simulink model "ScenarioLib"  (Simulink 7.8)
settings: Solver=ode45  StartTime=0.0  StopTime=10.0  RelTol=1e-3
undefined symbols (not defined in the file): sigbuilder_block
libraries: simulink x6, instrumentlib x4, utility x1, dspnetwork x1
settings Model: Creator=Zsolt  LastModifiedBy=jscott
settings DebuggingCC: FcnCallInpInsideContextMsg=Use local settings
settings HardwareCC: TargetIntDivRoundTo=Zero  TargetEndianess=LittleEndian  TargetHWDeviceType=MATLAB Host  ProdEqTarget=off
settings RTWCC: SystemTargetFile=rsim.tlc  TemplateMakefile=rsim_default_tmf  Description=Rapid Simulation Target  ProcessScript=rsim_make_rtw_hook
settings RSimTargetCC: TargetFunctionLibrary=ANSI_C  ERTMultiwordTypeDef=System defined  CodeExecutionProfiling=off  ERTMultiwordLength=256  IsPILTarget=off  EnableShiftOperators=on  PortableWordSizes=off

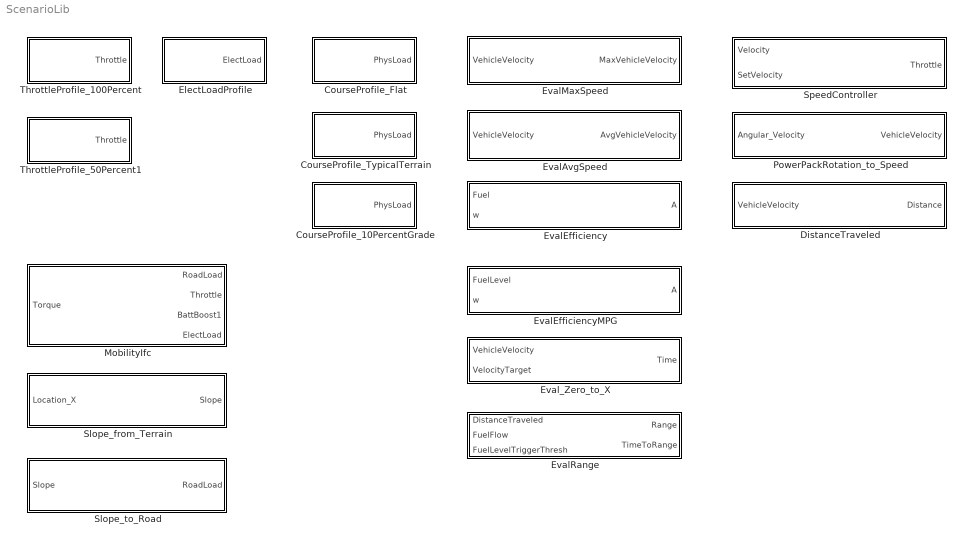
== system ScenarioLib ==
  CourseProfile_10PercentGrade : Subsystem
  CourseProfile_Flat : Subsystem
  CourseProfile_TypicalTerrain : Subsystem
  DistanceTraveled : Subsystem
  ElectLoadProfile : Subsystem
  EvalAvgSpeed : Subsystem
  EvalEfficiency : Subsystem
  EvalEfficiencyMPG : Subsystem
  EvalMaxSpeed : Subsystem
  EvalRange : Subsystem
  Eval_Zero_to_X : Subsystem
  MobilityIfc : Subsystem
  PowerPackRotation_to_Speed : Subsystem
  Slope_from_Terrain : Subsystem
  Slope_to_Road : Subsystem
  SpeedController : Subsystem
  ThrottleProfile_100Percent : Subsystem
  ThrottleProfile_50Percent1 : Subsystem

== system ScenarioLib/CourseProfile_10PercentGrade ==
  Flat : Subsystem  Tag=STV Subsys  LoadFcn=sigbuilder_block('load');  StartFcn=sigbuilder_block('start');  StopFcn=sigbuilder_block('stop');  ClipboardFcn=sigbuilder_block('clipboard');  mask(Sigbuilder block){}
      mask help: Create and generate interchangeable groups of signals whose waveforms are piecewise linear.
      mask init:
      | if ~strcmp(get_param(bdroot(gcbh),'SimulationStatus'),'stopped') tuvar = sigbuilder_block('maskInit'); end
      settings: CopyFcn=sigbuilder_block('copy');  DeleteFcn=sigbuilder_block('delete');  ModelCloseFcn=sigbuilder_block('modelClose');  PreSaveFcn=sigbuilder_block('preSave');  NameChangeFcn=sigbuilder_block('namechange');  OpenFcn=sigbuilder_block('open',[62.6897 69.5172 970.759 504 ]);  CloseFcn=sigbuilder_block('close');
      mask Display: plot(0,0,100,100,[10,10,40,40,10],[80,20,20,80,80],[40,10],[50,50], [40,27,10],[65,72,56],[40,25,25,10],[28,28,43,43]);
  PhysLoad : Outport
  wires:
  Flat/1(PhysLoad) -> PhysLoad/1

== system ScenarioLib/CourseProfile_Flat ==
  Flat : Subsystem  Tag=STV Subsys  LoadFcn=sigbuilder_block('load');  StartFcn=sigbuilder_block('start');  StopFcn=sigbuilder_block('stop');  ClipboardFcn=sigbuilder_block('clipboard');  mask(Sigbuilder block){}
      mask help: Create and generate interchangeable groups of signals whose waveforms are piecewise linear.
      mask init:
      | if ~strcmp(get_param(bdroot(gcbh),'SimulationStatus'),'stopped') tuvar = sigbuilder_block('maskInit'); end
      settings: CopyFcn=sigbuilder_block('copy');  DeleteFcn=sigbuilder_block('delete');  ModelCloseFcn=sigbuilder_block('modelClose');  PreSaveFcn=sigbuilder_block('preSave');  NameChangeFcn=sigbuilder_block('namechange');  OpenFcn=sigbuilder_block('open',[62.6897 69.5172 970.759 504 ]);  CloseFcn=sigbuilder_block('close');
      mask Display: plot(0,0,100,100,[10,10,40,40,10],[80,20,20,80,80],[40,10],[50,50], [40,27,10],[65,72,56],[40,25,25,10],[28,28,43,43]);
  PhysLoad : Outport
  wires:
  Flat/1(PhysLoad) -> PhysLoad/1

== system ScenarioLib/CourseProfile_TypicalTerrain ==
  TypicalTerrain : Subsystem  Tag=STV Subsys  LoadFcn=sigbuilder_block('load');  StartFcn=sigbuilder_block('start');  StopFcn=sigbuilder_block('stop');  ClipboardFcn=sigbuilder_block('clipboard');  mask(Sigbuilder block){}
      mask help: Create and generate interchangeable groups of signals whose waveforms are piecewise linear.
      mask init:
      | if ~strcmp(get_param(bdroot(gcbh),'SimulationStatus'),'stopped') tuvar = sigbuilder_block('maskInit'); end
      settings: CopyFcn=sigbuilder_block('copy');  DeleteFcn=sigbuilder_block('delete');  ModelCloseFcn=sigbuilder_block('modelClose');  PreSaveFcn=sigbuilder_block('preSave');  NameChangeFcn=sigbuilder_block('namechange');  OpenFcn=sigbuilder_block('open',[164.483 27.3103 970.138 504 ]);  CloseFcn=sigbuilder_block('close');
      mask Display: plot(0,0,100,100,[10,10,40,40,10],[80,20,20,80,80],[40,10],[50,50], [40,27,10],[65,72,56],[40,25,25,10],[28,28,43,43]);
  PhysLoad : Outport
  wires:
  TypicalTerrain/1(PhysLoad) -> PhysLoad/1

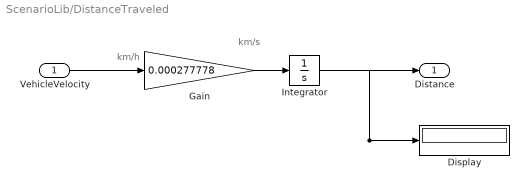
== system ScenarioLib/DistanceTraveled ==
  note: km/h
  note: km/s
  VehicleVelocity : Inport
  Display : Display
  Gain : Gain  Gain=0.000277778
  Integrator : Integrator
  Distance : Outport
  wires:
  VehicleVelocity/1 -> Gain/1
  Integrator/1 -> Distance/1, Display/1
  Gain/1 -> Integrator/1

== system ScenarioLib/ElectLoadProfile ==
  Elect_Load_Driver : Subsystem  Tag=STV Subsys  LoadFcn=sigbuilder_block('load');  StartFcn=sigbuilder_block('start');  StopFcn=sigbuilder_block('stop');  ClipboardFcn=sigbuilder_block('clipboard');  mask(Sigbuilder block){}
      mask help: Create and generate interchangeable groups of signals whose waveforms are piecewise linear.
      mask init:
      | if ~strcmp(get_param(bdroot(gcbh),'SimulationStatus'),'stopped') tuvar = sigbuilder_block('maskInit'); end
      settings: CopyFcn=sigbuilder_block('copy');  DeleteFcn=sigbuilder_block('delete');  ModelCloseFcn=sigbuilder_block('modelClose');  PreSaveFcn=sigbuilder_block('preSave');  NameChangeFcn=sigbuilder_block('namechange');  OpenFcn=sigbuilder_block('open',[164.483 24.8276 970.138 502.759 ]);  CloseFcn=sigbuilder_block('close');
      mask Display: plot(0,0,100,100,[10,10,40,40,10],[80,20,20,80,80],[40,10],[50,50], [40,27,10],[65,72,56],[40,25,25,10],[28,28,43,43]);
  ElectLoad : Outport
  wires:
  Elect_Load_Driver/1(Elect Load) -> ElectLoad/1

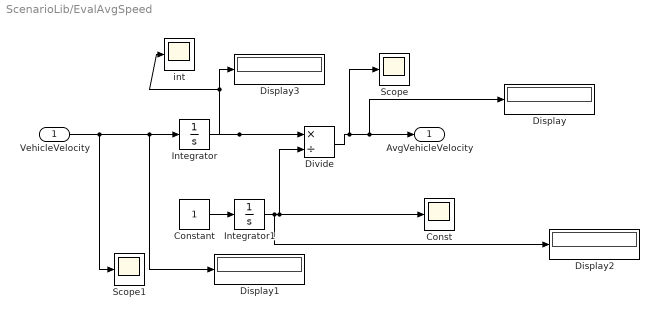
== system ScenarioLib/EvalAvgSpeed ==
  VehicleVelocity : Inport
  Const : Scope
      settings: YMin=250  YMax=4250
  Constant : Constant
  Display{,1..3} (4 alike) : Display
  Divide : Product  Inputs=*/
  Integrator : Integrator
  Integrator1 : Integrator  InitialCondition=0.001
  Scope : Scope
      settings: YMin=250  YMax=4250  SaveName=ScopeData2
  Scope1 : Scope
      settings: YMin=250  YMax=4250  SaveName=ScopeData3
  int : Scope
      settings: YMin=250  YMax=4250  SaveName=ScopeData4
  AvgVehicleVelocity : Outport
  wires:
  Divide/1 -> Scope/1, AvgVehicleVelocity/1, Display/1
  VehicleVelocity/1 -> Scope1/1, Display1/1, Integrator/1
  Constant/1 -> Integrator1/1
  Integrator/1 -> Divide/1, Display3/1, int/1
  Integrator1/1 -> Display2/1, Divide/2, Const/1

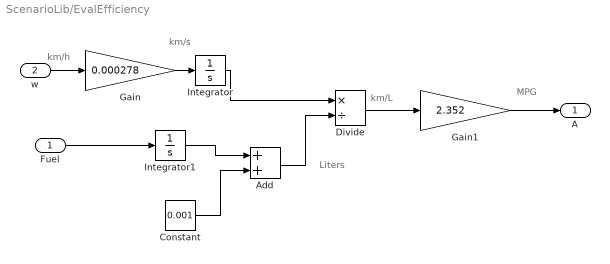
== system ScenarioLib/EvalEfficiency ==
  note: km/h
  note: km/s
  note: Liters
  note: km/L
  note: MPG
  Fuel : Inport
  w : Inport  Port=2
  Add : Sum
  Constant : Constant  Value=0.001
  Divide : Product  Inputs=*/
  Gain : Gain  Gain=0.000278
  Gain1 : Gain  Gain=2.352
  Integrator : Integrator
  Integrator1 : Integrator
  A : Outport
  wires:
  Integrator1/1 -> Add/1
  Constant/1 -> Add/2
  Fuel/1 -> Integrator1/1
  Add/1 -> Divide/2
  Integrator/1 -> Divide/1
  w/1 -> Gain/1
  Gain/1 -> Integrator/1
  Gain1/1 -> A/1
  Divide/1 -> Gain1/1

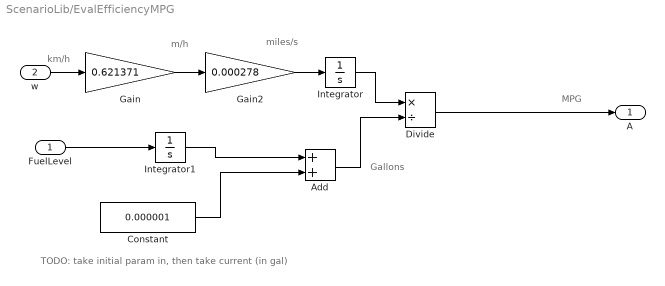
== system ScenarioLib/EvalEfficiencyMPG ==
  note: km/h
  note: m/h
  note: Gallons
  note: MPG
  note: TODO: take initial param in, then take current (in gal)
  note: miles/s
  FuelLevel : Inport
  w : Inport  Port=2
  Add : Sum
  Constant : Constant  Value=0.000001
  Divide : Product  Inputs=*/
  Gain : Gain  Gain=0.621371
  Gain2 : Gain  Gain=0.000278
  Integrator : Integrator
  Integrator1 : Integrator
  A : Outport
  wires:
  Integrator1/1 -> Add/1
  Constant/1 -> Add/2
  FuelLevel/1 -> Integrator1/1
  Add/1 -> Divide/2
  Integrator/1 -> Divide/1
  w/1 -> Gain/1
  Divide/1 -> A/1
  Gain2/1 -> Integrator/1
  Gain/1 -> Gain2/1

== system ScenarioLib/EvalMaxSpeed ==
  VehicleVelocity : Inport
  MinMax Running Resettable : simulink/Math Operations/MinMax Running Resettable  Function=max  vinit=0.0
  MaxVehicleVelocity : Outport
  wires:
  VehicleVelocity/1 -> MinMax Running Resettable/1
  MinMax Running Resettable/1 -> MaxVehicleVelocity/1

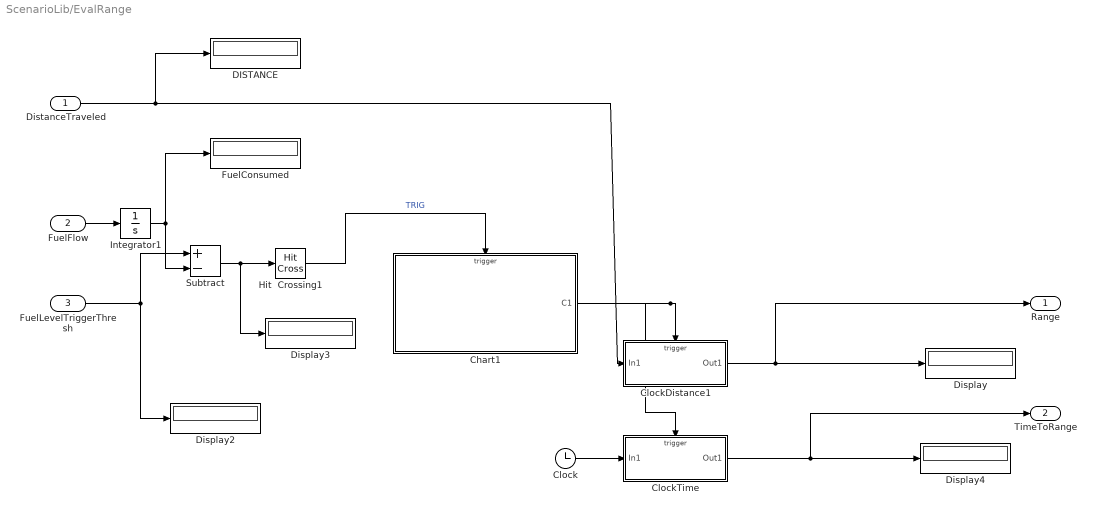
== system ScenarioLib/EvalRange ==
  DistanceTraveled : Inport
  FuelFlow : Inport  Port=2
  FuelLevelTriggerThresh : Inport  Port=3
  Chart1 : Stateflow chart  TreatAsAtomicUnit=on
  Clock : Clock
  ClockDistance1 : Subsystem  TreatAsAtomicUnit=on
  ClockTime : Subsystem  TreatAsAtomicUnit=on
  DISTANCE : Display
  Display{,2..4} (4 alike) : Display
  FuelConsumed : Display
  Hit  Crossing1 : HitCross  HitCrossingDirection=falling  ZeroCross=off
  Integrator1 : Integrator
  Subtract : Sum  Inputs=+-
  Range : Outport
  TimeToRange : Outport  Port=2
  wires:
  DistanceTraveled/1 -> ClockDistance1/1(In1), DISTANCE/1
  Hit  Crossing1/1 -> Chart1/Trigger  "TRIG"
  Chart1/1(C1) -> ClockDistance1/Trigger, ClockTime/Trigger
  ClockDistance1/1(Out1) -> Range/1, Display/1
  FuelFlow/1 -> Integrator1/1
  FuelLevelTriggerThresh/1 -> Display2/1, Subtract/1
  Subtract/1 -> Hit  Crossing1/1, Display3/1
  Clock/1 -> ClockTime/1(In1)
  ClockTime/1(Out1) -> TimeToRange/1, Display4/1
  Integrator1/1 -> FuelConsumed/1, Subtract/2

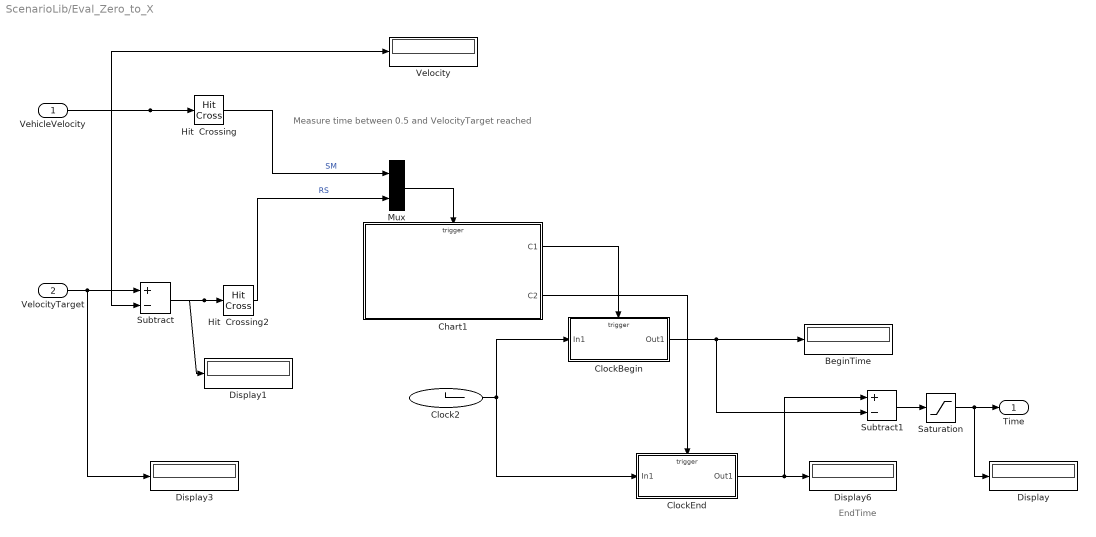
== system ScenarioLib/Eval_Zero_to_X ==
  note: EndTime
  note: Measure time between 0.5 and VelocityTarget reached
  VehicleVelocity : Inport
  VelocityTarget : Inport  Port=2
  BeginTime : Display
  Chart1 : Stateflow chart  TreatAsAtomicUnit=on
  Clock2 : Clock
  ClockBegin : Subsystem  TreatAsAtomicUnit=on
  ClockEnd : Subsystem  TreatAsAtomicUnit=on
  Display{,1,3,6} (4 alike) : Display
  Hit  Crossing : HitCross  HitCrossingOffset=0.5  HitCrossingDirection=rising
  Hit  Crossing2 : HitCross  HitCrossingDirection=falling  ZeroCross=off
  Mux : Mux  Inputs=2
  Saturation : Saturate  UpperLimit=10000000  LowerLimit=0.0  ZeroCross=off
  Subtract : Sum  Inputs=+-
  Subtract1 : Sum  Inputs=+-
  Velocity : Display
  Time : Outport
  wires:
  ClockBegin/1(Out1) -> BeginTime/1, Subtract1/2
  ClockEnd/1(Out1) -> Display6/1, Subtract1/1
  Chart1/2(C2) -> ClockEnd/Trigger
  Subtract/1 -> Display1/1, Hit  Crossing2/1
  VelocityTarget/1 -> Subtract/1, Display3/1
  Chart1/1(C1) -> ClockBegin/Trigger
  Hit  Crossing2/1 -> Mux/2  "RS"
  Hit  Crossing/1 -> Mux/1  "SM"
  Clock2/1 -> ClockBegin/1(In1), ClockEnd/1(In1)
  Mux/1 -> Chart1/Trigger
  VehicleVelocity/1 -> Hit  Crossing/1, Subtract/2, Velocity/1
  Subtract1/1 -> Saturation/1
  Saturation/1 -> Time/1, Display/1

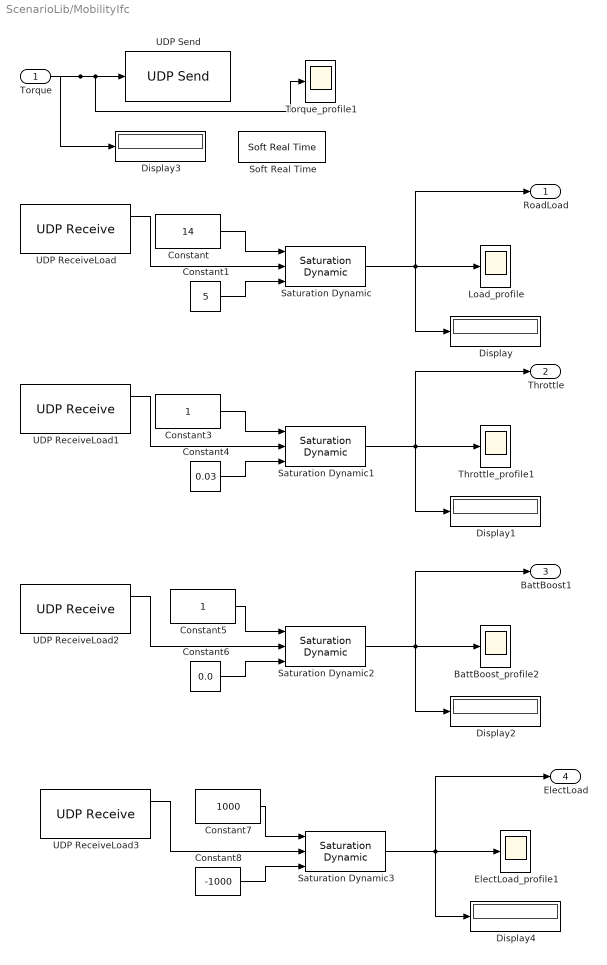
== system ScenarioLib/MobilityIfc ==
  Torque : Inport
  BattBoost_profile2 : Scope
      settings: TimeRange=500  YMin=0  YMax=150000  SaveName=ScopeData3
  Constant : Constant  Value=14
  Constant1 : Constant  Value=5
  Constant3 : Constant
  Constant4 : Constant  Value=0.03
  Constant5 : Constant
  Constant6 : Constant  Value=0.0
  Constant7 : Constant  Value=1000
  Constant8 : Constant  Value=-1000
  Display{,1..4} (5 alike) : Display
  ElectLoad_profile1 : Scope
      settings: TimeRange=500  YMin=0  YMax=150000  SaveName=ScopeData5
  Load_profile : Scope
      settings: TimeRange=500  YMin=0  YMax=150000
  Saturation Dynamic{,1..3} (4 alike) : simulink/Discontinuities/Saturation Dynamic  OutMin=[]  OutMax=[]  OutDataTypeStr=Inherit: Same as second input  OutDataType=fixdt(1, 16)  OutScaling=2^-10  DoSatur=off
  Soft Real Time : utility/Soft Real Time  x=1
  Throttle_profile1 : Scope
      settings: TimeRange=500  YMin=0  YMax=150000
  Torque_profile1 : Scope
      settings: TimeRange=100  YMin=0  YMax=150000  SaveName=ScopeData4
  UDP ReceiveLoad : instrumentlib/UDP Receive  Host=localhost  Port=9090  LocalPort=8090  DataSize=[1 1]  EnableBlockingMode=off  Timeout=10  SampleTime=0.08  DataType=double  ByteOrder=LittleEndian
  UDP ReceiveLoad1 : instrumentlib/UDP Receive  Host=localhost  Port=9090  LocalPort=8092  DataSize=[1 1]  EnableBlockingMode=off  Timeout=10  SampleTime=0.08  DataType=double  ByteOrder=LittleEndian
  UDP ReceiveLoad2 : instrumentlib/UDP Receive  Host=localhost  Port=9090  LocalPort=8093  DataSize=[1 1]  EnableBlockingMode=off  Timeout=10  SampleTime=0.08  DataType=double  ByteOrder=LittleEndian
  UDP ReceiveLoad3 : instrumentlib/UDP Receive  Host=localhost  Port=9090  LocalPort=8098  DataSize=[1 1]  EnableBlockingMode=off  Timeout=10  SampleTime=0.08  DataType=double  ByteOrder=LittleEndian
  UDP Send : dspnetwork/UDP Send  remoteURL='127.0.0.1'  remotePort=8094  localURL='0.0.0.0'  localPortSource=Automatically determine  localPort=-1  sampletime=-1  separateLengthPort=0
  RoadLoad : Outport
  Throttle : Outport  Port=2
  BattBoost1 : Outport  Port=3
  ElectLoad : Outport  Port=4
  wires:
  Constant/1 -> Saturation Dynamic/1
  Constant1/1 -> Saturation Dynamic/3
  Saturation Dynamic/1 -> Load_profile/1, Display/1, RoadLoad/1
  UDP ReceiveLoad/1 -> Saturation Dynamic/2
  Constant3/1 -> Saturation Dynamic1/1
  Constant4/1 -> Saturation Dynamic1/3
  Saturation Dynamic1/1 -> Throttle_profile1/1, Display1/1, Throttle/1
  UDP ReceiveLoad1/1 -> Saturation Dynamic1/2
  Constant5/1 -> Saturation Dynamic2/1
  Constant6/1 -> Saturation Dynamic2/3
  Saturation Dynamic2/1 -> BattBoost_profile2/1, Display2/1, BattBoost1/1
  UDP ReceiveLoad2/1 -> Saturation Dynamic2/2
  Torque/1 -> UDP Send/1, Torque_profile1/1, Display3/1
  Constant7/1 -> Saturation Dynamic3/1
  Constant8/1 -> Saturation Dynamic3/3
  Saturation Dynamic3/1 -> ElectLoad_profile1/1, Display4/1, ElectLoad/1
  UDP ReceiveLoad3/1 -> Saturation Dynamic3/2

== system ScenarioLib/PowerPackRotation_to_Speed ==
  Angular_Velocity : Inport
  Gain : Gain  Gain=0.3
  VehicleVelocity : Outport
  wires:
  Gain/1 -> VehicleVelocity/1
  Angular_Velocity/1 -> Gain/1

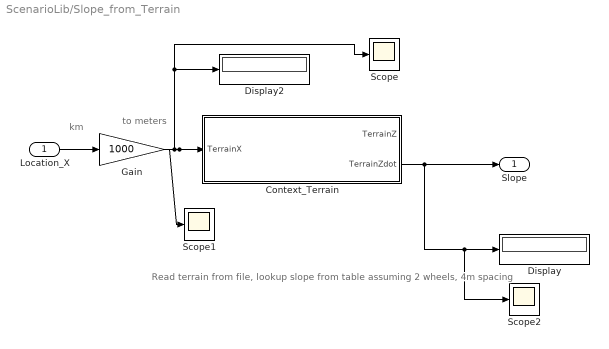
== system ScenarioLib/Slope_from_Terrain ==
  note: Read terrain from file, lookup slope from table
      |  assuming 2 wheels, 4m spacing
  note: km
  note: to meters
  Location_X : Inport
  Context_Terrain : Subsystem  mask(Context Model Terrain for Fuel Efficiency){TerrainFilename=terrain.txt, Use_Old_Terrain=off, Input0_Height=0, Input_QueryDist=off, Output_Height_CkBx=on, Output_Slope_CkBx=on, TerrainLength=20000}
      mask prompts: TerrainFilename "Terrain Filename"; Use_Old_Terrain "Use Existing Terrain"; Input0_Height "Initial Terrain Height"; Input_QueryDist "Query with Distance Traveled"; Output_Height_CkBx "Height_Output"; Output_Slope_CkBx "Slope_Output"; TerrainLength "Desired Terrain Length"
      mask help: Generates a sample terrain from a Probability Density Function fit of US CONUS DEM data. The DEM data was sampled at 90 meter increments, consequently the data establishes long wavelength changes in slope suitable for the study of gross elevation changes on a system design.
      mask init:
      | ThisBlock = gcb;
      | % verify the existence of terrain file
      | if and(strcmp(Use_Old_Terrain, 'off'), ...
      |         ~exist(TerrainFilename, 'file'))
      |     msgbox(['Terrain filename: ', TerrainFilename, ...
      |         ' does not exist. Setting "Use Existing ', ...
      |         'Terrain" checkbox to create new instance', ...
      |         '.  Remember to un-check it after this run.']);
      |     set_param(ThisBlock, 'Use_Old_Terrain', 'off');
      | end
      | % test for terrain synthesis
      | if strcmp(Use_Old_Terrain, 'on')
      |     % load up the existing terrain data
      |     x = load(TerrainFilename, 'ascii');
      |     % terrain data is stored in orthogonal coordinates
      |     % calculate the slope data and load it up
      |     SignedSlope = [diff(x(:,2))./diff(x(:,1)),0];
      | else
      |     % generate some new terrain
      |     npts = ceil(TerrainLength/92/2)*2;
      |     x = zeros(npts,2);
      |     x(:,1) = [0:92:(npts-1)*92]'; % distance in meters
      |     % form a slope array
      |     Slope = 0.037*(log(rand(npts,1))+log(rand(npts,1)));
      |     SignedSlope = sign(rand(npts,1)-0.5).*Slope;
      |     % Form the elevation array
      |     Elevation = [0; diff(x(:,1))].*SignedSlope;
      |     x(:,2) = cumsum(Elevation)'; % distance in meters
      |     % save the synthesized terrain
      |     save(TerrainFilename, 'x', '-ascii')
      | end
      | % adjust for terrain query method
      | if strcmp(Input_QueryDist, 'on')
      |     % set for distance traveled
      |     terrain_in = [0, cumsum(sqrt(diff(x(:,1)).^2 + ...
      |         diff(x(:,2)).^2))];
      | else
      |     terrain_in = x(:,1)';
      | end
      | terrain_out = x(:,2)';
      | % load up the terrain data into the lookup tables
      | set_param([ThisBlock, '/Terrain Height'], ...
      |     'InputValues', ['[', num2str(terrain_in), ']'], ...
      |     'OutputValues', ['[', num2str(terrain_out), ']']);
      | set_param([ThisBlock, '/Terrain Heightdot'], ...
      |     'InputValues', ['[', num2str(terrain_in), ']'], ...
      |     'OutputValues', ['[', num2str(SignedSlope(2:end)'), ' 0]']);
      mask Help:
      | Copyright (c) 2012, BAE Systems.
      | Developed with the sponsorship of the Defense Advanced Research Projects Agency (DARPA).
      | 
      | Permission is hereby granted, free of charge, to any person obtaining a copy of this data,
      | including any software or models in source or binary form, as well as any drawings,
      | specifications, and documentation (collectively "the Data"), to deal in the Data without restriction,
      | including without limitation the rights to use, copy, modify, merge, publish, distribute, sublicense,
      | and/or sell copies of the Data, and to permit persons to whom the Data is furnished to do so,
      | subject to the following conditions:
      | 
      | The above copyright notice and this permission notice shall be included in all copies or substantial
      | portions of the Data.
      | 
      | THE DATA IS PROVIDED "AS IS", WITHOUT WARRANTY OF ANY KIND, EXPRESS OR IMPLIED, INCLUDING
      | BUT NOT LIMITED TO THE WARRANTIES OF MERCHANTABILITY, FITNESS FOR A PARTICULAR PURPOSE
      | AND NONINFRINGEMENT. IN NO EVENT SHALL THE AUTHORS, SPONSORS, DEVELOPERS, CONTRIBUTORS,
      | OR COPYRIGHT HOLDERS BE LIABLE FOR ANY CLAIM, DAMAGES OR OTHER LIABILITY, WHETHER IN AN
      | ACTION OF CONTRACT, TORT OR OTHERWISE, ARISING FROM, OUT OF OR IN CONNECTION WITH THE
      | DATA OR THE USE OR OTHER DEALINGS IN THE DATA.
      mask CallbackString:
      | ThisBlock = gcb;
      | Use_Old_Terrain = get_param(ThisBlock, 'Use_Old_Terrain');
      | TerrainFilename = get_param(ThisBlock, 'TerrainFilename');
      | % file must exist for terrain use
      | if strcmp(Use_Old_Terrain,'on')
      |     if ~exist(TerrainFilename, 'file')
      |         msgbox(['Terrain filename: ', TerrainFilename, ...
      |             ' does not exist. Setting "Use Existing ', ...
      |             'Terrain" checkbox to create new instance', ...
      |             '.  Remember to un-check it after this run.']);
      |         % uncheck the Use Old Terrain chkbox
      |         set_param(ThisBlock, 'Use_Old_Terrain', 'off');
      |     end
      | end|ThisBlock = gcb;
      | Use_Old_Terrain = get_param(ThisBlock, 'Use_Old_Terrain');
      | TerrainFilename = get_param(ThisBlock, 'TerrainFilename');
      | % file must exist for terrain use
      | if strcmp(Use_Old_Terrain,'on')
      |     if ~exist(TerrainFilename, 'file')
      |         msgbox(['Terrain filename: ', TerrainFilename, ...
      |             ' does not exist. Setting "Use Existing ', ...
      |             'Terrain" checkbox to create new instance', ...
      |             '.  Change "Terrain Filename" to existing', ...
      |             ' file before setting this checkbox.']);
      |         % uncheck the Use Old Terrain chkbox
      |         set_param(ThisBlock, 'Use_Old_Terrain', 'off');
      |     else
      |         % load up the terrain file and change the length parameter
      |         tmp = load(TerrainFilename, 'ascii');
      |         TerrainLength = max(tmp(:,1));
      |         % change the terrain length parameter
      |         set_param(ThisBlock, 'TerrainLength', num2str(TerrainLength));
      |     end
      | end|ThisBlock = gcb;
      | Input0_Height = get_param(ThisBlock, 'Input0_Height');
      | % set the constant offset block
      | set_param([ThisBlock, '/Ref_Height'], 'Value', num2str(Input0_Height));||ThisBlock = gcb;
      | Output_Slope_CkBx = get_param(ThisBlock, 'Output_Slope_CkBx');
      | Output_Height_CkBx = get_param(ThisBlock, 'Output_Height_CkBx');
      | % check what number to use for the output port
      | if strcmp(Output_Height_CkBx, 'on')
      |     if strcmp(Output_Slope_CkBx, 'on')
      |         % set the output port number to 2
      |         set_param([ThisBlock, '/TerrainZdot'], ...
      |             'Port', '2');
      |     end
      |     % replace with output block
      |     replace_block([ThisBlock, '/TerrainZ'], ...
      |         'Terminator', 'built-in/Outport', ...
      |         'noprompt')
      | else
      |     % replace with Terminator
      |     replace_block([ThisBlock, '/TerrainZ'], ...
      |         'Outport', 'built-in/Terminator', ...
      |         'noprompt')
      | end
      | |ThisBlock = gcb;
      | Output_Slope_CkBx = get_param(ThisBlock, 'Output_Slope_CkBx');
      | Output_Height_CkBx = get_param(ThisBlock, 'Output_Height_CkBx');
      | % check what number to use for the output port
      | if strcmp(Output_Height_CkBx, 'on')
      |     % set the output port number to 2
      |     SlopePortNum = '2';
      | else
      |     SlopePortNum = '1';
      | end
      | % set or add the appropriate outputs
      | if strcmp(Output_Slope_CkBx, 'on')
      |     % replace with output block
      |     replace_block([ThisBlock, '/TerrainZdot'], ...
      |         'Terminator', 'built-in/Outport', ...
      |         'noprompt')
      |     set_param([ThisBlock, '/TerrainZdot'], ...
      |         'Port', SlopePortNum);
      | else
      |     % replace with Terminator
      |     replace_block([ThisBlock, '/TerrainZdot'], ...
      |         'Outport', 'built-in/Terminator', ...
      |         'noprompt')
      | end|ThisBlock = gcb;
      | TerrainLength = get_param(ThisBlock, 'TerrainLength');
      | % verify that the length is positive
      | if str2num(TerrainLength)<=0
      |     msgbox(['Desired terrain length needs to be greater than zero.  ', ...
      |         'Setting the value to 1000 meters.']);
      |     set_param(ThisBlock, 'TerrainLength', num2str(1000));
      | end
      mask TabNameString: Primary,Primary,Primary,Set-up,Set-up,Set-up,Set-up
  Display : Display
  Display2 : Display
  Gain : Gain  Gain=1000
  Scope : Scope
      settings: SaveName=ScopeData12
  Scope1 : Scope
      settings: SaveName=ScopeData13
  Scope2 : Scope
      settings: SaveName=ScopeData14
  Slope : Outport
  wires:
  Location_X/1 -> Gain/1
  Context_Terrain/2(TerrainZdot) -> Slope/1, Display/1, Scope2/1
  Gain/1 -> Display2/1, Scope/1, Context_Terrain/1(TerrainX), Scope1/1

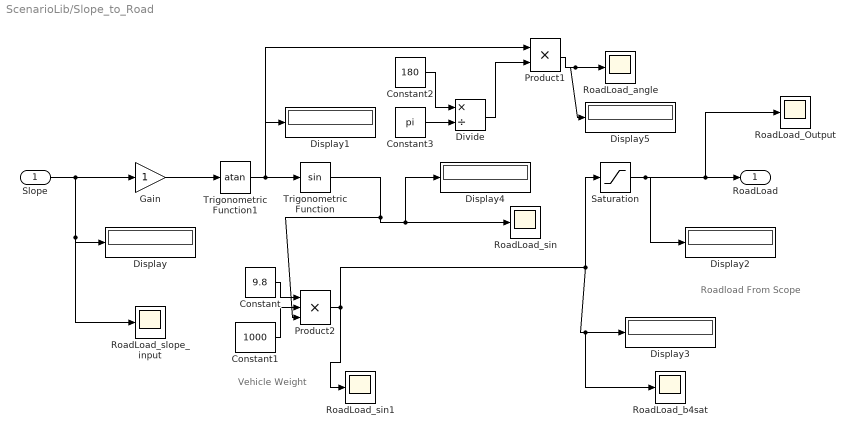
== system ScenarioLib/Slope_to_Road ==
  note: Vehicle Weight
  note: Roadload From Scope
  Slope : Inport
  Constant : Constant  Value=9.8
  Constant1 : Constant  Value=1000
  Constant2 : Constant  Value=180
  Constant3 : Constant  Value=pi
  Display{,1..5} (6 alike) : Display
  Divide : Product  Inputs=*/
  Gain : Gain
  Product1 : Product  RndMeth=Zero
  Product2 : Product  Inputs=3  RndMeth=Zero
  RoadLoad_Output : Scope
      settings: YMin=250  YMax=4250  SaveName=ScopeData7
  RoadLoad_angle : Scope
      settings: YMin=250  YMax=4250  SaveName=ScopeData8
  RoadLoad_b4sat : Scope
      settings: YMin=250  YMax=4250  SaveName=ScopeData6
  RoadLoad_sin : Scope
      settings: YMin=250  YMax=4250  SaveName=ScopeData9
  RoadLoad_sin1 : Scope
      settings: YMin=250  YMax=4250  SaveName=ScopeData10
  RoadLoad_slope_input : Scope
      settings: YMin=250  YMax=4250  SaveName=ScopeData11
  Saturation : Saturate  UpperLimit=20000  LowerLimit=0
  Trigonometric Function : Trigonometry
  Trigonometric Function1 : Trigonometry  Operator=atan
  RoadLoad : Outport
  wires:
  Trigonometric Function/1 -> RoadLoad_sin/1, Display4/1, Product2/3
  Trigonometric Function1/1 -> Trigonometric Function/1, Display1/1, Product1/1
  Saturation/1 -> Display2/1, RoadLoad/1, RoadLoad_Output/1
  Gain/1 -> Trigonometric Function1/1
  Slope/1 -> Display/1, RoadLoad_slope_input/1, Gain/1
  Constant2/1 -> Divide/1
  Constant3/1 -> Divide/2
  Divide/1 -> Product1/2
  Product1/1 -> RoadLoad_angle/1, Display5/1
  Constant/1 -> Product2/1
  Constant1/1 -> Product2/2
  Product2/1 -> RoadLoad_sin1/1, RoadLoad_b4sat/1, Display3/1, Saturation/1

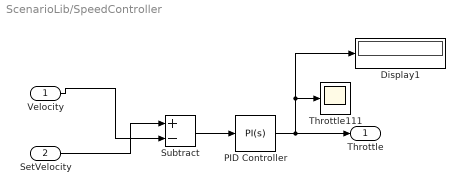
== system ScenarioLib/SpeedController ==
  Velocity : Inport
  SetVelocity : Inport  Port=2
  Display1 : Display
  PID Controller : simulink/Continuous/PID Controller  Controller=PI  TimeDomain=Continuous-time  SampleTime=1  IntegratorMethod=Forward Euler  FilterMethod=Forward Euler  Form=Parallel  P=0.01  I=0.1  D=0  N=100  InitialConditionSource=internal  InitialConditionForIntegrator=0  InitialConditionForFilter=0  ExternalReset=none  LimitOutput=on  UpperSaturationLimit=1  LowerSaturationLimit=0  LinearizeAsGain=off  AntiWindupMode=clamping  Kb=1  TrackingMode=off  Kt=1  PParamMin=[]  PParamMax=[]  IParamMin=[]  IParamMax=[]  DParamMin=[]  DParamMax=[]  NParamMin=[]  NParamMax=[]  KbParamMin=[]  KbParamMax=[]  KtParamMin=[]  KtParamMax=[]  POutMin=[]  POutMax=[]  IOutMin=[]  IOutMax=[]  DOutMin=[]  DOutMax=[]  NOutMin=[]  NOutMax=[]  KbOutMin=[]  KbOutMax=[]  KtOutMin=[]  KtOutMax=[]  IntegratorOutMin=[]  IntegratorOutMax=[]  FilterOutMin=[]  FilterOutMax=[]  SumOutMin=[]  SumOutMax=[]  SumI1OutMin=[]  SumI1OutMax=[]  SumI2OutMin=[]  SumI2OutMax=[]  SumI3OutMin=[]  SumI3OutMax=[]  SumDOutMin=[]  SumDOutMax=[]  SaturationOutMin=[]  SaturationOutMax=[]  IntegratorContinuousStateAttributes=''  IntegratorStateMustResolveToSignalObject=off  IntegratorRTWStateStorageClass=Auto  FilterContinuousStateAttributes=''  FilterStateMustResolveToSignalObject=off  FilterRTWStateStorageClass=Auto
  Subtract : Sum  Inputs=+-
  Throttle111 : Scope
      settings: TimeRange=100  YMin=-3  YMax=8
  Throttle : Outport
  wires:
  Velocity/1 -> Subtract/2
  SetVelocity/1 -> Subtract/1
  Subtract/1 -> PID Controller/1
  PID Controller/1 -> Throttle/1, Throttle111/1, Display1/1

== system ScenarioLib/ThrottleProfile_100Percent ==
  Differential driver1 : Subsystem  Tag=STV Subsys  LoadFcn=sigbuilder_block('load');  StartFcn=sigbuilder_block('start');  StopFcn=sigbuilder_block('stop');  ClipboardFcn=sigbuilder_block('clipboard');  mask(Sigbuilder block){}
      mask help: Create and generate interchangeable groups of signals whose waveforms are piecewise linear.
      mask init:
      | if ~strcmp(get_param(bdroot(gcbh),'SimulationStatus'),'stopped') tuvar = sigbuilder_block('maskInit'); end
      settings: CopyFcn=sigbuilder_block('copy');  DeleteFcn=sigbuilder_block('delete');  ModelCloseFcn=sigbuilder_block('modelClose');  PreSaveFcn=sigbuilder_block('preSave');  NameChangeFcn=sigbuilder_block('namechange');  OpenFcn=sigbuilder_block('open',[164.483 24.2069 970.138 502.759 ]);  CloseFcn=sigbuilder_block('close');
      mask Display: plot(0,0,100,100,[10,10,40,40,10],[80,20,20,80,80],[40,10],[50,50], [40,27,10],[65,72,56],[40,25,25,10],[28,28,43,43]);
  Throttle : Outport
  wires:
  Differential driver1/1(Throttle) -> Throttle/1

== system ScenarioLib/ThrottleProfile_50Percent1 ==
  Differential driver1 : Subsystem  Tag=STV Subsys  LoadFcn=sigbuilder_block('load');  StartFcn=sigbuilder_block('start');  StopFcn=sigbuilder_block('stop');  ClipboardFcn=sigbuilder_block('clipboard');  mask(Sigbuilder block){}
      mask help: Create and generate interchangeable groups of signals whose waveforms are piecewise linear.
      mask init:
      | if ~strcmp(get_param(bdroot(gcbh),'SimulationStatus'),'stopped') tuvar = sigbuilder_block('maskInit'); end
      settings: CopyFcn=sigbuilder_block('copy');  DeleteFcn=sigbuilder_block('delete');  ModelCloseFcn=sigbuilder_block('modelClose');  PreSaveFcn=sigbuilder_block('preSave');  NameChangeFcn=sigbuilder_block('namechange');  OpenFcn=sigbuilder_block('open',[164.483 25.4483 970.138 502.759 ]);  CloseFcn=sigbuilder_block('close');
      mask Display: plot(0,0,100,100,[10,10,40,40,10],[80,20,20,80,80],[40,10],[50,50], [40,27,10],[65,72,56],[40,25,25,10],[28,28,43,43]);
  Throttle : Outport
  wires:
  Differential driver1/1(Throttle) -> Throttle/1

== system ScenarioLib/CourseProfile_10PercentGrade/Flat ==
  Demux : Demux  Tag=STV Demux  Outputs=1
  FromWs : FromWorkspace  Tag=STV FromWs  VariableName=tuvar  SampleTime=0  SigBuilderData=DataTag0  VnvData=DataTag1
      SigBuilderData=|
      | common.afterFinalStr = 'Extrapolate'
      | common.sampleTime = 0
      | dataSet.timeRange = [0 100]
      | dataSet.name = 'Group 1'
      | sbobj.Groups.Name = 'Group 1'
      | sbobj.Groups.Signals.Name = 'PhysLoad'
      | sbobj.Groups.Signals.XData = [0 100]
      | sbobj.Groups.Signals.YData = [9 9]
  PhysLoad : Outport  Tag=STV Outport
  wires:
  FromWs/1 -> Demux/1
  Demux/1 -> PhysLoad/1

== system ScenarioLib/CourseProfile_Flat/Flat ==
  Demux : Demux  Tag=STV Demux  Outputs=1
  FromWs : FromWorkspace  Tag=STV FromWs  VariableName=tuvar  SampleTime=0  SigBuilderData=DataTag2  VnvData=DataTag3
      SigBuilderData=|
      | common.afterFinalStr = 'Extrapolate'
      | common.sampleTime = 0
      | dataSet.timeRange = [0 100]
      | dataSet.name = 'Group 1'
      | sbobj.Groups.Name = 'Group 1'
      | sbobj.Groups.Signals.Name = 'PhysLoad'
      | sbobj.Groups.Signals.XData = [0 100]
      | sbobj.Groups.Signals.YData = [7 7]
  PhysLoad : Outport  Tag=STV Outport
  wires:
  FromWs/1 -> Demux/1
  Demux/1 -> PhysLoad/1

== system ScenarioLib/CourseProfile_TypicalTerrain/TypicalTerrain ==
  Demux : Demux  Tag=STV Demux  Outputs=1
  FromWs : FromWorkspace  Tag=STV FromWs  VariableName=tuvar  SampleTime=0  SigBuilderData=DataTag4  VnvData=DataTag5
      SigBuilderData=|
      | common.afterFinalStr = 'Extrapolate'
      | common.sampleTime = 0
      | dataSet.timeRange = [0 100]
      | dataSet.name = 'Group 1'
      | sbobj.Groups.Name = 'Group 1'
      | sbobj.Groups.Signals.Name = 'PhysLoad'
      | sbobj.Groups.Signals.XData = [0 14.9 14.9 20 40.1 44.8 44.8 55.2 55.2 60.2 75 80.1 100]
      | sbobj.Groups.Signals.YData = [6.98 6.98 7 8 8 7 6.98 6.98 7 12 12 6 6]
  PhysLoad : Outport  Tag=STV Outport
  wires:
  FromWs/1 -> Demux/1
  Demux/1 -> PhysLoad/1

== system ScenarioLib/ElectLoadProfile/Elect_Load_Driver ==
  Demux : Demux  Tag=STV Demux  Outputs=1
  FromWs : FromWorkspace  Tag=STV FromWs  VariableName=tuvar  SampleTime=0  SigBuilderData=DataTag6  VnvData=DataTag7
      SigBuilderData=|
      | common.afterFinalStr = 'Extrapolate'
      | common.sampleTime = 0
      | dataSet.timeRange = [0 100]
      | dataSet.name = 'Group 1'
      | sbobj.Groups.Name = 'Group 1'
      | sbobj.Groups.Signals.Name = 'Elect Load'
      | sbobj.Groups.Signals.XData = [0 36.8 70 100]
      | sbobj.Groups.Signals.YData = [45000 45000 45000 45000]
  Elect Load : Outport  Tag=STV Outport
  wires:
  Demux/1 -> Elect Load/1
  FromWs/1 -> Demux/1

== system ScenarioLib/EvalRange/ClockDistance1 ==
  In1 : Inport
  Trigger : TriggerPort
  Out1 : Outport
  wires:
  In1/1 -> Out1/1

== system ScenarioLib/EvalRange/ClockTime ==
  In1 : Inport
  Trigger : TriggerPort
  Out1 : Outport
  wires:
  In1/1 -> Out1/1

== system ScenarioLib/Eval_Zero_to_X/ClockBegin ==
  In1 : Inport
  Trigger : TriggerPort  ZeroCross=off
  Out1 : Outport
  wires:
  In1/1 -> Out1/1

== system ScenarioLib/Eval_Zero_to_X/ClockEnd ==
  In1 : Inport
  Trigger : TriggerPort  ZeroCross=off
  Display1 : Display
  Display4 : Display
  Out1 : Outport
  wires:
  In1/1 -> Display1/1, Out1/1, Display4/1

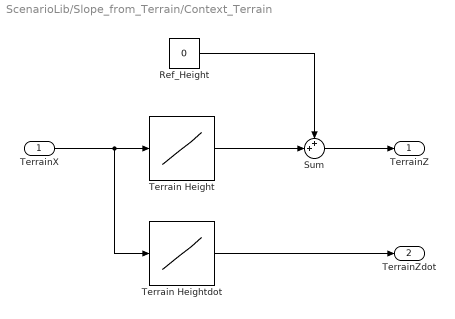
== system ScenarioLib/Slope_from_Terrain/Context_Terrain ==
  TerrainX : Inport
  Ref_Height : Constant  Value=0
  Sum : Sum  Inputs=++|
  Terrain Height : Lookup  InputValues="[0     92    184    276    368    460    552    644    736    828    920   1012   1104   1196   1288   1380   1472   1564   1656   1748   1840   1932   2024   2116   2208   2300   2392   2484   2576   2668   2760   2852   2944   3036   3128   3220   3312   3404   3496   3588   3680   3772   3864   3956   4048   4140   4232   4324   4416   4508   4600   4692   4784   4876   4968   5060   5152   5244   5336   5428   5520   5612   5704   5796   5888   5980   6072   6164   6256   6348   6440   6532   6624   6716   6808   6900   6992   7084   7176   7268   7360   7452   7544   7636   7728   7820   7912   8004   8096   8188   8280   8372   8464   8556   8648   8740   8832   8924   9016   9108   9200   9292   9384   9476   9568   9660   9752   9844   9936  10028  10120  10212  10304  10396  10488  10580  10672  10764  10856  10948  11040  11132  11224  11316  11408  11500  11592  11684  11776  11868  11960  12052  12144  12236  12328  12420  12512  12604  12696  12788  12880  12972  13064  13156  13248  13340  13432  13524  13616  13708  13800  13892  13984  14076  14168  14260  14352  14444  14536  14628  14720  14812  14904  14996  15088  15180  15272  15364  15456  15548  15640  15732  15824  15916  16008  16100  16192  16284  16376  16468  16560  16652  16744  16836  16928  17020  17112  17204  17296  17388  17480  17572  17664  17756  17848  17940  18032  18124  18216  18308  18400  18492  18584  18676  18768  18860  18952  19044  19136  19228  19320  19412  19504  19596  19688  19780  19872  19964]"  Table="[0     -9.314944     -5.562551     -1.156475       9.23678      3.717174     -7.659609     -5.137529      11.27193      6.507215      4.459013      9.575071      6.014597      2.910176      19.94266      14.35199       17.6497      25.43216      14.65231      9.530139      10.71504     -5.756384       -10.602     -20.27741     -14.00759     -11.50117     -4.690092     -8.331273       4.80455      14.34541      7.956171     -2.376044      7.731915      15.34933      29.82479      21.98818      24.49084      26.84709      21.53546      22.07317      5.959201      1.762234      11.62041      23.40871       15.7005      11.72827     -8.771383     -10.31011     -9.233403      -10.3356     -6.389186     -1.363018      4.045249     -11.28514     -21.11314     -27.39307     -30.51009      -21.9419     -24.51197     -18.29983     -28.50731     -29.27494      -31.3831     -27.07037     -22.22009     -31.90313     -35.20714     -37.62854     -39.95424     -51.48427     -54.62386     -62.30588     -56.79432      -64.2904     -61.02905     -54.79159     -62.87352     -58.78004     -49.33228     -56.33841     -48.87135     -44.42724       -39.316     -29.80613     -16.60827     -23.71835     -15.07092     -10.17167      6.067621      20.13795      16.48602      26.43369      20.77044       18.7834       10.5384      7.568621      17.58537      21.22515     -1.916436      4.692964     -18.01321     -32.45471      -40.9008      -33.4166     -43.34797      -32.0867     -29.40181     -29.03084     -34.95883     -40.93541     -48.96575     -52.32144     -49.37016     -56.81128     -46.60174      -51.7956     -58.47259      -74.3929     -83.44873     -88.10723     -87.65346     -81.14376     -100.7226     -98.42691     -86.21443     -84.53464      -81.5961     -88.76046     -95.40497     -102.8105     -97.19393     -97.60672     -98.66833     -101.8972     -107.1151     -102.3355     -102.8846     -100.0581     -106.8214     -113.7196     -115.4501     -110.6915      -111.983     -100.3742     -98.09824     -101.3618     -107.3375     -96.28654     -112.0812     -119.9887     -115.0492     -110.8503     -100.2118     -96.09958     -88.84551      -95.7629     -89.79504     -110.0952     -109.1879     -116.0464     -112.8563     -118.5628     -127.8729     -122.9934     -111.2789     -84.03303     -74.60717     -67.82772     -62.42258     -64.93466     -70.29886     -77.62836     -69.42843     -70.46315     -66.48355     -68.93639     -71.57928     -66.76528      -74.3386     -77.49291     -83.70008     -92.51708     -99.38857     -90.99984     -85.91861     -81.29975     -82.89232      -88.7242     -69.64851     -66.45377     -70.95428     -73.22223     -75.65342       -68.497     -90.06632     -97.22218     -88.53176     -85.81575     -60.14914      -63.1671     -66.51149     -42.90914     -55.92294     -62.72644     -58.95999     -48.59351     -66.60906     -75.02329     -88.26968     -89.18308     -82.08746      -77.4986     -87.88137     -103.8336      -117.588     -112.1593     -117.2383     -121.0257]"  LookUpMeth=Interpolation-Use End Values
  Terrain Heightdot : Lookup  InputValues="[0     92    184    276    368    460    552    644    736    828    920   1012   1104   1196   1288   1380   1472   1564   1656   1748   1840   1932   2024   2116   2208   2300   2392   2484   2576   2668   2760   2852   2944   3036   3128   3220   3312   3404   3496   3588   3680   3772   3864   3956   4048   4140   4232   4324   4416   4508   4600   4692   4784   4876   4968   5060   5152   5244   5336   5428   5520   5612   5704   5796   5888   5980   6072   6164   6256   6348   6440   6532   6624   6716   6808   6900   6992   7084   7176   7268   7360   7452   7544   7636   7728   7820   7912   8004   8096   8188   8280   8372   8464   8556   8648   8740   8832   8924   9016   9108   9200   9292   9384   9476   9568   9660   9752   9844   9936  10028  10120  10212  10304  10396  10488  10580  10672  10764  10856  10948  11040  11132  11224  11316  11408  11500  11592  11684  11776  11868  11960  12052  12144  12236  12328  12420  12512  12604  12696  12788  12880  12972  13064  13156  13248  13340  13432  13524  13616  13708  13800  13892  13984  14076  14168  14260  14352  14444  14536  14628  14720  14812  14904  14996  15088  15180  15272  15364  15456  15548  15640  15732  15824  15916  16008  16100  16192  16284  16376  16468  16560  16652  16744  16836  16928  17020  17112  17204  17296  17388  17480  17572  17664  17756  17848  17940  18032  18124  18216  18308  18400  18492  18584  18676  18768  18860  18952  19044  19136  19228  19320  19412  19504  19596  19688  19780  19872  19964]"  Table="[-0.10125    0.040787    0.047892     0.11297   -0.059996    -0.12366    0.027414     0.17836    -0.05179   -0.022263    0.055609   -0.038701   -0.033744     0.18514   -0.060768    0.035845    0.084592    -0.11717   -0.055676    0.012879    -0.17904    -0.05267    -0.10517     0.06815    0.027244    0.074033   -0.039578     0.14278     0.10371   -0.069448    -0.11231     0.10987    0.082798     0.15734   -0.085181    0.027203    0.025611   -0.057735   0.0058446    -0.17515   -0.045619     0.10715     0.12813   -0.083785   -0.043176    -0.22282   -0.016725    0.011703    -0.01198    0.042896    0.054632    0.058786    -0.16663    -0.10683    -0.06826   -0.033881    0.093133   -0.027936    0.067523    -0.11095  -0.0083438   -0.022915    0.046877     0.05272    -0.10525   -0.035913    -0.02632   -0.025279    -0.12533   -0.034126     -0.0835    0.059908   -0.081479    0.035449    0.067798   -0.087847    0.044494     0.10269   -0.076154    0.081164    0.048306    0.055557     0.10337     0.14345   -0.077283    0.093994    0.053253     0.17651     0.15294   -0.039695     0.10813   -0.061557   -0.021598    -0.08962    -0.03228     0.10888    0.039563    -0.25154    0.071841    -0.24681    -0.15697   -0.091805     0.08135    -0.10795     0.12241    0.029184   0.0040323   -0.064435   -0.064963   -0.087286   -0.036475    0.032079   -0.080882     0.11097   -0.056455   -0.072576    -0.17305   -0.098433   -0.050636   0.0049323    0.070758    -0.21281    0.024953     0.13274    0.018259    0.031941   -0.077873   -0.072223   -0.080495     0.06105  -0.0044868   -0.011539   -0.035096   -0.056716    0.051952  -0.0059691    0.030723   -0.073513   -0.074981    -0.01881    0.051724   -0.014038     0.12618    0.024738   -0.035474   -0.064953     0.12012    -0.17168   -0.085951     0.05369     0.04564     0.11564    0.044698    0.078849   -0.075189    0.064868    -0.22065   0.0098625   -0.074549    0.034675   -0.062027     -0.1012    0.053038     0.12733     0.29615     0.10246     0.07369    0.058752   -0.027305   -0.058307   -0.079668     0.08913   -0.011247    0.043257   -0.026661   -0.028727    0.052326   -0.082319   -0.034286   -0.067469   -0.095837    -0.07469    0.091182    0.055231    0.050205   -0.017311    -0.06339     0.20734    0.034725   -0.048919   -0.024652   -0.026426    0.077787    -0.23445   -0.077781    0.094461    0.029522     0.27898   -0.032804   -0.036352     0.25655    -0.14145   -0.073951     0.04094     0.11268    -0.19582   -0.091459    -0.14398  -0.0099283    0.077126    0.049879    -0.11286    -0.17339     -0.1495    0.059008   -0.055207   -0.041167 0]"  LookUpMeth=Use Input Below
  TerrainZ : Outport
  TerrainZdot : Outport  Port=2
  wires:
  TerrainX/1 -> Terrain Height/1, Terrain Heightdot/1
  Terrain Height/1 -> Sum/2
  Ref_Height/1 -> Sum/1
  Sum/1 -> TerrainZ/1
  Terrain Heightdot/1 -> TerrainZdot/1

== system ScenarioLib/ThrottleProfile_100Percent/Differential driver1 ==
  Demux : Demux  Tag=STV Demux  Outputs=1
  FromWs : FromWorkspace  Tag=STV FromWs  VariableName=tuvar  SampleTime=0  SigBuilderData=DataTag8  VnvData=DataTag9
      SigBuilderData=|
      | common.afterFinalStr = 'Extrapolate'
      | common.sampleTime = 0
      | dataSet.timeRange = [0 100]
      | dataSet.name = 'Group 1'
      | sbobj.Groups.Name = 'Group 1'
      | sbobj.Groups.Signals.Name = 'Throttle'
      | sbobj.Groups.Signals.XData = [0 4 36.8 70 100]
      | sbobj.Groups.Signals.YData = [1 1 1 1 1]
  Throttle : Outport  Tag=STV Outport
  wires:
  Demux/1 -> Throttle/1
  FromWs/1 -> Demux/1

== system ScenarioLib/ThrottleProfile_50Percent1/Differential driver1 ==
  Demux : Demux  Tag=STV Demux  Outputs=1
  FromWs : FromWorkspace  Tag=STV FromWs  VariableName=tuvar  SampleTime=0  SigBuilderData=DataTag10  VnvData=DataTag11
      SigBuilderData=|
      | common.afterFinalStr = 'Extrapolate'
      | common.sampleTime = 0
      | dataSet.timeRange = [0 100]
      | dataSet.name = 'Group 1'
      | sbobj.Groups.Name = 'Group 1'
      | sbobj.Groups.Signals.Name = 'Throttle'
      | sbobj.Groups.Signals.XData = [0 4 36.8 70 100]
      | sbobj.Groups.Signals.YData = [0.5 0.5 0.5 0.5 0.5]
  Throttle : Outport  Tag=STV Outport
  wires:
  Demux/1 -> Throttle/1
  FromWs/1 -> Demux/1

== stateflow chart EvalRange/Chart1 ==
  settings: executeAtInitialization=1
  state WAIT_FOR_FUEL_LEVEL_THRESH
  state MEASURE_DIST
  WAIT_FOR_FUEL_LEVEL_THRESH -> MEASURE_DIST : TRIG/C1
  (default) -> WAIT_FOR_FUEL_LEVEL_THRESH
  events: TRIG input RISING_EDGE_EVENT; C1 output EITHER_EDGE_EVENT

== stateflow chart Eval_Zero_to_X/Chart1 ==
  settings: sampleTime=1  executeAtInitialization=1
  state WAIT_ON_VEH_MOVEMENT
  state MEASURE_TIME
  state END
  WAIT_ON_VEH_MOVEMENT -> MEASURE_TIME : SM/C1
  MEASURE_TIME -> END : RS/C2
  (default) -> WAIT_ON_VEH_MOVEMENT
  events: SM input RISING_EDGE_EVENT; RS input RISING_EDGE_EVENT; C1 output EITHER_EDGE_EVENT; C2 output EITHER_EDGE_EVENT
